simulink model "exampleModel_bus_axi_w_4ptavg"  (R2017b)
settings: Solver=VariableStepAuto  StartTime=0.0  StopTime=10e-5  RelTol=1e-3
PreLoadFcn:
  | setup
values from neighbouring files (symbols this model uses):
  axiClk = 156.25e6    (= 156250000)    [setup.m]    (also in setup_exampleModel_bus_axi_simulink.m; setup_exampleModel_bus_axi_simulink_lcls2.m; setup_lcls2_pcav.m; sysgen_signal.m)
  cav1p1_addr = 204    [setup_exampleModel_bus_axi_simulink.m]    (also in setup_exampleModel_bus_axi_simulink_lcls2.m; setup_lcls2_pcav.m; sysgen_signal.m)
  cav1p2_addr = cav1p1_addr * 2    (= 408)    [setup_exampleModel_bus_axi_simulink.m]    (also in setup_exampleModel_bus_axi_simulink_lcls2.m; setup_lcls2_pcav.m; sysgen_signal.m)
  cav2p1_addr = cav1p1_addr * 3    (= 612)    [setup_exampleModel_bus_axi_simulink.m]    (also in setup_exampleModel_bus_axi_simulink_lcls2.m; setup_lcls2_pcav.m; sysgen_signal.m)
  cav2p2_addr = cav1p1_addr * 4    (= 816)    [setup_exampleModel_bus_axi_simulink.m]    (also in setup_exampleModel_bus_axi_simulink_lcls2.m; setup_lcls2_pcav.m; sysgen_signal.m)
  Fadc = Fs/interleavedChannels    (= 29750000)    [setup.m]    (also in setup_exampleModel_bus_axi_simulink.m = 357000000; setup_exampleModel_bus_axi_simulink_lcls2.m = 351000000; setup_lcls2_pcav.m = 357000000; sysgen_signal.m = 357000000)
  fir_lpf = fir1(15, w_lpf)    [setup_exampleModel_bus_axi_simulink.m]    (also in setup_exampleModel_bus_axi_simulink_lcls2.m; setup_lcls2_pcav.m)
  Fproc = 204e6    (= 204000000)    [setup_exampleModel_bus_axi_simulink.m]    (also in setup_exampleModel_bus_axi_simulink_lcls2.m = 200571400; setup_lcls2_pcav.m; sysgen_signal.m)
  Fsig = Fproc/12    (= 17000000)    [setup_exampleModel_bus_axi_simulink.m]    (also in setup_exampleModel_bus_axi_simulink_lcls2.m = 16714283.3333; setup_lcls2_pcav.m)
  Tadc = 1/fadc    (= 2.80112044818e-09)    [cavity_signal.m]    (also in setup_exampleModel_bus_axi_simulink.m; setup_exampleModel_bus_axi_simulink_lcls2.m = 2.849002849e-09; setup_lcls2_pcav.m; setup_pcav_simulink.m)
undefined symbols (not defined in the file or in its folder): AXI4, Lite
libraries: xbsIndex_r4 x2870, llrf_lib x10, simulink x3
(part 8 of 15)

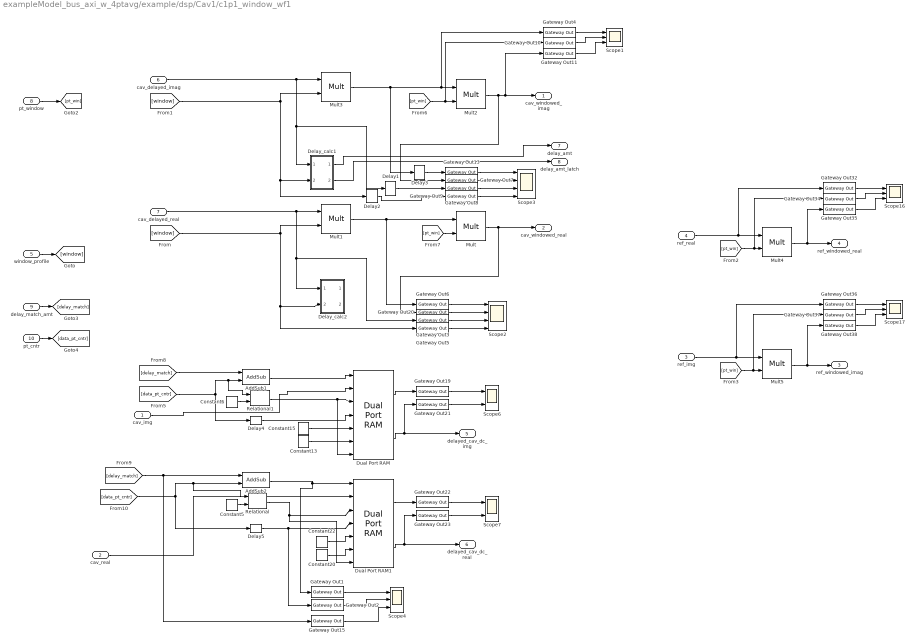
== system exampleModel_bus_axi_w_4ptavg/example/dsp/Cav1/c1p1_window_wf1  ==
  cav_img : Inport
  cav_real : Inport  Port=2
  ref_img : Inport  Port=3
  ref_real : Inport  Port=4
  window_profile : Inport  Port=5
  cav_delayed_imag : Inport  Port=6
  cav_delayed_real : Inport  Port=7
  pt_window : Inport  Port=8
  delay_match_amt : Inport  Port=9
  pt_cntr : Inport  Port=10
  AddSub1 : xbsIndex_r4/AddSub  mode=Addition  use_carryin=off  use_carryout=off  en=off  latency=1  precision=User Defined  arith_type=Unsigned  n_bits=16  bin_pt=0  quantization=Truncate  overflow=Wrap  use_behavioral_HDL=off  hw_selection=Fabric  pipelined=off  dbl_ovrd=off  block_type=addsub
  AddSub2 : xbsIndex_r4/AddSub  mode=Addition  use_carryin=off  use_carryout=off  en=off  latency=1  precision=User Defined  arith_type=Unsigned  n_bits=16  bin_pt=0  quantization=Truncate  overflow=Wrap  use_behavioral_HDL=off  hw_selection=Fabric  pipelined=off  dbl_ovrd=off  block_type=addsub
  Constant13 : xbsIndex_r4/Constant  const=1  gui_display_data_type=Boolean  arith_type=Boolean  n_bits=16  bin_pt=14  preci_type=Single  exp_width=8  frac_width=24  explicit_period=off  period=1  equ=P=C  opselect=C  inp2=PCIN>>17  opr=+  inp1=P  carry=CIN  dbl_ovrd=off  block_type=constant
  Constant{5..6,15,22} (4 alike) : xbsIndex_r4/Constant  const=0  gui_display_data_type=Fixed-point  arith_type=Signed (2's comp)  n_bits=18  bin_pt=16  preci_type=Single  exp_width=8  frac_width=24  explicit_period=off  period=1  equ=P=C  opselect=C  inp2=PCIN>>17  opr=+  inp1=P  carry=CIN  dbl_ovrd=off  block_type=constant
  Constant20 : xbsIndex_r4/Constant  const=1  gui_display_data_type=Boolean  arith_type=Boolean  n_bits=16  bin_pt=14  preci_type=Single  exp_width=8  frac_width=24  explicit_period=off  period=1  equ=P=C  opselect=C  inp2=PCIN>>17  opr=+  inp1=P  carry=CIN  dbl_ovrd=off  block_type=constant
  Delay1 : xbsIndex_r4/Delay  rst=off  infoeditControl=Selection of Reset will increase slice count due to use of real FFs and instead of SRLs  en=off  latency=6  reg_retiming=off  dbl_ovrd=off  block_type=delay
  Delay2 : xbsIndex_r4/Delay  rst=off  infoeditControl=Selection of Reset will increase slice count due to use of real FFs and instead of SRLs  en=off  latency=6  reg_retiming=off  dbl_ovrd=off  block_type=delay
  Delay3 : xbsIndex_r4/Delay  rst=off  infoeditControl=Selection of Reset will increase slice count due to use of real FFs and instead of SRLs  en=off  latency=3  reg_retiming=off  dbl_ovrd=off  block_type=delay
  Delay4 : xbsIndex_r4/Delay  rst=off  infoeditControl=Selection of Reset will increase slice count due to use of real FFs and instead of SRLs  en=off  latency=1  reg_retiming=off  dbl_ovrd=off  block_type=delay
  Delay5 : xbsIndex_r4/Delay  rst=off  infoeditControl=Selection of Reset will increase slice count due to use of real FFs and instead of SRLs  en=off  latency=1  reg_retiming=off  dbl_ovrd=off  block_type=delay
  Delay_calc1 : Subsystem
  Delay_calc2 : Subsystem
  Dual Port RAM : xbsIndex_r4/Dual Port RAM  depth=2^16  initVector=zeros(2^16,1)  distributed_mem=Block RAM  init_a=0  init_b=0  rst_a=off  rst_b=off  en_a=off  en_b=on  latency=1  write_mode_A=Read After Write  write_mode_B=Read Before Write  optimize=Area  dbl_ovrd=off  block_type=dpram
  Dual Port RAM1 : xbsIndex_r4/Dual Port RAM  depth=2^16  initVector=zeros(2^16,1)  distributed_mem=Block RAM  init_a=0  init_b=0  rst_a=off  rst_b=off  en_a=off  en_b=on  latency=1  write_mode_A=Read After Write  write_mode_B=Read Before Write  optimize=Area  dbl_ovrd=off  block_type=dpram
  Gateway Out{1..3,5..9,13,15,19..23} (15 alike) : xbsIndex_r4/Gateway Out  inherit_from_input=off  hdl_port=off  rows=1  columns=1  UseAsDAC=off  DACChannel='1'  interface=None  automatic_assignment=on  address_offset=hex2dec('00')  intf_name=''  intf_description=''  timing_constraint=None  locs_specified=off  LOCs={}  io_standard={}  block_type=gatewayout
  Gateway Out{4,10..11,32,34..38} (9 alike) : xbsIndex_r4/Gateway Out  inherit_from_input=off  hdl_port=on  rows=1  columns=1  UseAsDAC=off  DACChannel='1'  interface=None  automatic_assignment=on  address_offset=hex2dec('00')  intf_name=''  intf_description=''  timing_constraint=None  locs_specified=off  LOCs={}  io_standard={}  block_type=gatewayout
  Mult{,2,4..5} (4 alike) : xbsIndex_r4/Mult  precision=User Defined  arith_type="Signed  (2's comp)"  n_bits=18  bin_pt=16  quantization=Truncate  overflow=Wrap  en=off  latency=3  use_behavioral_HDL=off  opt=Speed  use_embedded=on  optimum_pipeline=off  pipeline=on  dbl_ovrd=off  use_rpm=on  placement_style=Triangular  block_type=mult
  Mult1 : xbsIndex_r4/Mult  precision=User Defined  arith_type="Signed  (2's comp)"  n_bits=18  bin_pt=17  quantization=Truncate  overflow=Wrap  en=off  latency=3  use_behavioral_HDL=off  opt=Speed  use_embedded=on  optimum_pipeline=off  pipeline=on  dbl_ovrd=off  use_rpm=on  placement_style=Triangular  block_type=mult
  Mult3 : xbsIndex_r4/Mult  precision=User Defined  arith_type="Signed  (2's comp)"  n_bits=18  bin_pt=17  quantization=Truncate  overflow=Wrap  en=off  latency=3  use_behavioral_HDL=off  opt=Speed  use_embedded=on  optimum_pipeline=off  pipeline=on  dbl_ovrd=off  use_rpm=on  placement_style=Triangular  block_type=mult
  Relational : xbsIndex_r4/Relational  mode=a>b  op_type=Bool  en=off  latency=1  dbl_ovrd=off  block_type=relational
  Relational1 : xbsIndex_r4/Relational  mode=a>b  op_type=Bool  en=off  latency=1  dbl_ovrd=off  block_type=relational
  Scope{1,4,16..17} (4 alike) : Scope  NumInputPorts=3
  Scope2 : Scope  NumInputPorts=4
  Scope3 : Scope  NumInputPorts=4
  Scope6 : Scope  NumInputPorts=2
  Scope7 : Scope  NumInputPorts=2
  cav_windowed_imag : Outport
  cav_windowed_real : Outport  Port=2
  ref_windowed_imag : Outport  Port=3
  ref_windowed_real : Outport  Port=4
  delayed_cav_dc_img : Outport  Port=5
  delayed_cav_dc_real : Outport  Port=6
  delay_amt : Outport  Port=7
  delay_amt_latch : Outport  Port=8
  wires:
  cav_real/1 -> Dual Port RAM1/2
  Relational/1 -> Dual Port RAM1/7, Dual Port RAM1/3
  Mult2/1 -> Gateway Out11/1, cav_windowed_imag/1, Gateway Out7/1
  Gateway Out23/1 -> Scope7/2
  Gateway Out21/1 -> Scope6/2
  Dual Port RAM1/1 -> Gateway Out22/1
  [data_pt_cntr] -> Relational1/1, AddSub1/2, Delay4/1
  Constant15/1 -> Dual Port RAM/5
  Gateway Out20/1 -> Scope2/2
  AddSub1/1 -> Dual Port RAM/1
  [pt_win] -> Gateway Out10/1, Mult2/2
  Gateway Out8/1 -> Scope3/3
  Gateway Out3/1 -> Scope2/3
  Constant13/1 -> Dual Port RAM/6
  Mult/1 -> cav_windowed_real/1, Gateway Out20/1
  cav_delayed_imag/1 -> Mult3/1, Delay_calc1/1(wav), Delay1/1
  [delay_match] -> Gateway Out15/1, AddSub2/1
  Gateway Out19/1 -> Scope6/1
  Gateway Out9/1 -> Scope3/4
  [data_pt_cntr] -> Delay5/1, Relational/1, AddSub2/2
  Dual Port RAM/1 -> Gateway Out19/1
  Gateway Out22/1 -> Scope7/1
  [window] -> Delay_calc1/2(win), Delay2/1, Mult3/2
  [window] -> Mult1/2, Delay_calc2/2(win), Gateway Out5/1
  cav_delayed_real/1 -> Delay_calc2/1(wav), Gateway Out3/1, Mult1/1
  Constant20/1 -> Dual Port RAM1/6
  Mult1/1 -> Gateway Out6/1, Mult/1
  Constant22/1 -> Dual Port RAM1/5
  Gateway Out6/1 -> Scope2/1
  Gateway Out13/1 -> Scope3/1
  [delay_match] -> AddSub1/1
  Gateway Out5/1 -> Scope2/4
  Gateway Out7/1 -> Scope3/2
  [pt_win] -> Mult/2
  Gateway Out35/1 -> Scope16/3
  ref_img/1 -> Gateway Out36/1, Mult5/1
  [pt_win] -> Gateway Out37/1, Mult5/2
  [pt_win] -> Gateway Out34/1, Mult4/2
  ref_real/1 -> Gateway Out32/1, Mult4/1
  Mult5/1 -> ref_windowed_imag/1, Gateway Out38/1
  Gateway Out38/1 -> Scope17/3
  Gateway Out36/1 -> Scope17/1
  Gateway Out32/1 -> Scope16/1
  Gateway Out34/1 -> Scope16/2
  Mult4/1 -> ref_windowed_real/1, Gateway Out35/1
  Gateway Out37/1 -> Scope17/2
  window_profile/1 -> [window]
  Delay_calc1/1(delay_amt) -> delay_amt/1
  pt_window/1 -> [pt_win]
  delay_match_amt/1 -> [delay_match]
  pt_cntr/1 -> [data_pt_cntr]
  Mult3/1 -> Delay3/1, Gateway Out4/1, Mult2/1
  Delay1/1 -> Gateway Out8/1
  Delay2/1 -> Gateway Out9/1
  Delay3/1 -> Gateway Out13/1
  Delay_calc1/2(delay_fb_latch) -> delay_amt_latch/1
  Gateway Out1/1 -> Scope4/1
  Gateway Out2/1 -> Scope4/2
  AddSub2/1 -> Gateway Out1/1, Dual Port RAM1/1
  cav_img/1 -> Dual Port RAM/2
  Delay4/1 -> Dual Port RAM/4
  Gateway Out15/1 -> Scope4/3
  Delay5/1 -> Gateway Out2/1, Dual Port RAM1/4
  Dual Port RAM1/2 -> delayed_cav_dc_real/1, Gateway Out23/1
  Dual Port RAM/2 -> delayed_cav_dc_img/1, Gateway Out21/1
  Constant5/1 -> Relational/2
  Constant6/1 -> Relational1/2
  Relational1/1 -> Dual Port RAM/7, Dual Port RAM/3
  Gateway Out10/1 -> Scope1/2
  Gateway Out4/1 -> Scope1/1
  Gateway Out11/1 -> Scope1/3

== system exampleModel_bus_axi_w_4ptavg/example/dsp/Cav1/c1p2_freq_err_module ==
  imag : Inport
  real : Inport  Port=2
  flo_window : Inport  Port=3
  reset : Inport  Port=4
  CORDIC 6.0 2 : xbsIndex_r4/CORDIC 6.0   functional_selection=Translate  architectural_configuration=Parallel  pipelining_mode=Maximum  data_format=SignedFraction  phase_format=Radians  input_width=18  output_width=18  round_mode=Truncate  iterations=0  precision=0  compensation_scaling=No_Scale_Compensation  coarse_rotation=on  aclken=off  aresetn=off  out_tready=off  cartesian_has_tuser=off  cartesian_has_tlast=off  cartesian_tuser_width=1  phase_has_tuser=off  phase_has_tlast=off  phase_tuser_width=1  out_tlast_behv=Null  flow_control=NonBlocking  optimize_goal=Resources  trim_axipin_name=on  simulation_type=hybrid_sim  simulation_model=sysgen:cordic_v6_0  data_path_portlist={'s_axis_cartesian_tdata_imag', 's_axis_cartesian_tdata_real', 's_axis_phase_tdata_phase', 'm_axis_dout_tdata_imag', 'm_axis_dout_tdata_real', 'm_axis_dout_tdata_phase','m_axis_dout_tdata'}  ip_name=CORDIC  ip_version=6.0  dsptool_ready=true  ipcore_usecache=true  ipcore_useipmodelcache=true  wrapper_available=true  port_translation_map={ 'aclken' => 'en', 'aresetn' => 'rst' }  block_type=cordic_v6_0
      settings: infoedit=CORDIC 6.0
  Clock Enable Probe4 : xbsIndex_r4/Clock Enable Probe  inherit_constraints=on  block_type=ceprobe
      settings: infoedit="Clock enable extractor.  Produces a Boolean output that mirrors the hardware clock enable associated with the input sample rate.<br><br>Hardware notes: in hardware this block costs nothing."
  Down Sample5 : xbsIndex_r4/Down Sample  sample_ratio=12  sample_phase="Last Value of Frame  (most efficient)"  en=off  rst=off  latency=1  dbl_ovrd=off  block_type=dsamp
  Gateway Out{1..3,38,41,53} (6 alike) : xbsIndex_r4/Gateway Out  inherit_from_input=off  hdl_port=off  rows=1  columns=1  UseAsDAC=off  DACChannel='1'  interface=None  automatic_assignment=on  address_offset=hex2dec('00')  intf_name=''  intf_description=''  timing_constraint=None  locs_specified=off  LOCs={}  io_standard={}  block_type=gatewayout
  Gateway Out44 : xbsIndex_r4/Gateway Out  inherit_from_input=off  hdl_port=on  rows=1  columns=1  UseAsDAC=off  DACChannel='1'  interface=None  automatic_assignment=on  address_offset=hex2dec('00')  intf_name=''  intf_description=''  timing_constraint=None  locs_specified=off  LOCs={}  io_standard={}  block_type=gatewayout
  Gateway Out46 : xbsIndex_r4/Gateway Out  inherit_from_input=off  hdl_port=on  rows=1  columns=1  UseAsDAC=off  DACChannel='1'  interface=None  automatic_assignment=on  address_offset=hex2dec('00')  intf_name=''  intf_description=''  timing_constraint=None  locs_specified=off  LOCs={}  io_standard={}  block_type=gatewayout
  Mult3 : xbsIndex_r4/Mult  precision=User Defined  arith_type="Signed  (2's comp)"  n_bits=18  bin_pt=15  quantization=Truncate  overflow=Saturate  en=off  latency=3  use_behavioral_HDL=off  opt=Speed  use_embedded=on  optimum_pipeline=off  pipeline=on  dbl_ovrd=off  use_rpm=on  placement_style=Triangular  block_type=mult
  Scope1 : Scope  NumInputPorts=3
  Scope21 : Scope  NumInputPorts=3
  Scope22 : Scope  NumInputPorts=2
  freq_err1 : Subsystem
  NCO_err_fb : Outport
  freq_err : Outport  Port=2
  wires:
  [c1p2_pt_cntr] -> Gateway Out41/1
  Down Sample5/1 -> CORDIC 6.0 2/1
  Gateway Out38/1 -> Scope21/2
  reset/1 -> freq_err1/3(reset)
  Clock Enable Probe4/1 -> Down Sample5/1
  CORDIC 6.0 2/2 -> freq_err1/1(raw_phase), Gateway Out38/1
  real/1 -> CORDIC 6.0 2/3, Gateway Out44/1
  imag/1 -> CORDIC 6.0 2/2, Clock Enable Probe4/1, Gateway Out46/1
  flo_window/1 -> Gateway Out2/1, Mult3/2, freq_err1/2(window)
  Gateway Out44/1 -> Scope22/2
  Gateway Out53/1 -> Scope21/1
  Gateway Out41/1 -> Scope21/3
  freq_err1/1(NCO_err) -> NCO_err_fb/1
  Gateway Out46/1 -> Scope22/1
  freq_err1/2(freq_err) -> freq_err/1
  Mult3/1 -> Gateway Out1/1
  Gateway Out1/1 -> Scope1/3
  Gateway Out3/1 -> Scope1/1
  Gateway Out2/1 -> Scope1/2
  CORDIC 6.0 2/3 -> Gateway Out3/1, Mult3/1, Gateway Out53/1

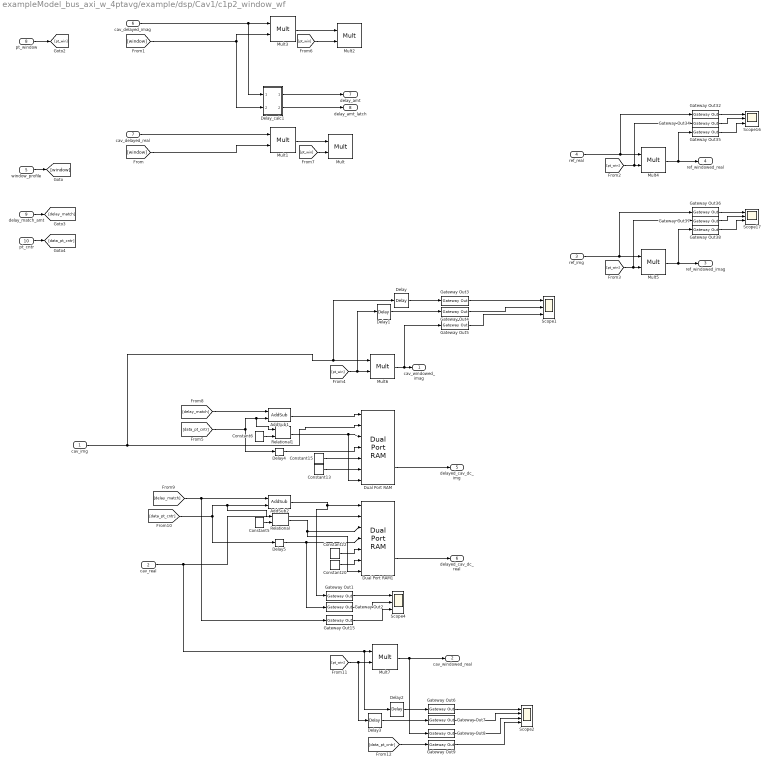
== system exampleModel_bus_axi_w_4ptavg/example/dsp/Cav1/c1p2_window_wf ==
  cav_img : Inport
  cav_real : Inport  Port=2
  ref_img : Inport  Port=3
  ref_real : Inport  Port=4
  window_profile : Inport  Port=5
  cav_delayed_imag : Inport  Port=6
  cav_delayed_real : Inport  Port=7
  pt_window : Inport  Port=8
  delay_match_amt : Inport  Port=9
  pt_cntr : Inport  Port=10
  AddSub1 : xbsIndex_r4/AddSub  mode=Addition  use_carryin=off  use_carryout=off  en=off  latency=1  precision=User Defined  arith_type=Unsigned  n_bits=16  bin_pt=0  quantization=Truncate  overflow=Wrap  use_behavioral_HDL=off  hw_selection=Fabric  pipelined=off  dbl_ovrd=off  block_type=addsub
  AddSub2 : xbsIndex_r4/AddSub  mode=Addition  use_carryin=off  use_carryout=off  en=off  latency=1  precision=User Defined  arith_type=Unsigned  n_bits=16  bin_pt=0  quantization=Truncate  overflow=Wrap  use_behavioral_HDL=off  hw_selection=Fabric  pipelined=off  dbl_ovrd=off  block_type=addsub
  Constant13 : xbsIndex_r4/Constant  const=1  gui_display_data_type=Boolean  arith_type=Boolean  n_bits=16  bin_pt=14  preci_type=Single  exp_width=8  frac_width=24  explicit_period=off  period=1  equ=P=C  opselect=C  inp2=PCIN>>17  opr=+  inp1=P  carry=CIN  dbl_ovrd=off  block_type=constant
  Constant{5..6,15,22} (4 alike) : xbsIndex_r4/Constant  const=0  gui_display_data_type=Fixed-point  arith_type=Signed (2's comp)  n_bits=18  bin_pt=16  preci_type=Single  exp_width=8  frac_width=24  explicit_period=off  period=1  equ=P=C  opselect=C  inp2=PCIN>>17  opr=+  inp1=P  carry=CIN  dbl_ovrd=off  block_type=constant
  Constant20 : xbsIndex_r4/Constant  const=1  gui_display_data_type=Boolean  arith_type=Boolean  n_bits=16  bin_pt=14  preci_type=Single  exp_width=8  frac_width=24  explicit_period=off  period=1  equ=P=C  opselect=C  inp2=PCIN>>17  opr=+  inp1=P  carry=CIN  dbl_ovrd=off  block_type=constant
  Delay{,1..3} (4 alike) : xbsIndex_r4/Delay  rst=off  infoeditControl=Selection of Reset will increase slice count due to use of real FFs and instead of SRLs  en=off  latency=3  reg_retiming=off  dbl_ovrd=off  block_type=delay
  Delay4 : xbsIndex_r4/Delay  rst=off  infoeditControl=Selection of Reset will increase slice count due to use of real FFs and instead of SRLs  en=off  latency=1  reg_retiming=off  dbl_ovrd=off  block_type=delay
  Delay5 : xbsIndex_r4/Delay  rst=off  infoeditControl=Selection of Reset will increase slice count due to use of real FFs and instead of SRLs  en=off  latency=1  reg_retiming=off  dbl_ovrd=off  block_type=delay
  Delay_calc1 : Subsystem
  Dual Port RAM : xbsIndex_r4/Dual Port RAM  depth=2^16  initVector=zeros(2^16,1)  distributed_mem=Block RAM  init_a=0  init_b=0  rst_a=off  rst_b=off  en_a=off  en_b=on  latency=1  write_mode_A=Read After Write  write_mode_B=Read Before Write  optimize=Area  dbl_ovrd=off  block_type=dpram
  Dual Port RAM1 : xbsIndex_r4/Dual Port RAM  depth=2^16  initVector=zeros(2^16,1)  distributed_mem=Block RAM  init_a=0  init_b=0  rst_a=off  rst_b=off  en_a=off  en_b=on  latency=1  write_mode_A=Read After Write  write_mode_B=Read Before Write  optimize=Area  dbl_ovrd=off  block_type=dpram
  Gateway Out{1..9,15} (10 alike) : xbsIndex_r4/Gateway Out  inherit_from_input=off  hdl_port=off  rows=1  columns=1  UseAsDAC=off  DACChannel='1'  interface=None  automatic_assignment=on  address_offset=hex2dec('00')  intf_name=''  intf_description=''  timing_constraint=None  locs_specified=off  LOCs={}  io_standard={}  block_type=gatewayout
  Gateway Out{32,34..38} (6 alike) : xbsIndex_r4/Gateway Out  inherit_from_input=off  hdl_port=on  rows=1  columns=1  UseAsDAC=off  DACChannel='1'  interface=None  automatic_assignment=on  address_offset=hex2dec('00')  intf_name=''  intf_description=''  timing_constraint=None  locs_specified=off  LOCs={}  io_standard={}  block_type=gatewayout
  Mult{,2,4..7} (6 alike) : xbsIndex_r4/Mult  precision=User Defined  arith_type="Signed  (2's comp)"  n_bits=18  bin_pt=16  quantization=Truncate  overflow=Wrap  en=off  latency=3  use_behavioral_HDL=off  opt=Speed  use_embedded=on  optimum_pipeline=off  pipeline=on  dbl_ovrd=off  use_rpm=on  placement_style=Triangular  block_type=mult
  Mult1 : xbsIndex_r4/Mult  precision=User Defined  arith_type="Signed  (2's comp)"  n_bits=18  bin_pt=17  quantization=Truncate  overflow=Wrap  en=off  latency=3  use_behavioral_HDL=off  opt=Speed  use_embedded=on  optimum_pipeline=off  pipeline=on  dbl_ovrd=off  use_rpm=on  placement_style=Triangular  block_type=mult
  Mult3 : xbsIndex_r4/Mult  precision=Full  arith_type="Signed  (2's comp)"  n_bits=18  bin_pt=17  quantization=Truncate  overflow=Wrap  en=off  latency=3  use_behavioral_HDL=off  opt=Speed  use_embedded=on  optimum_pipeline=off  pipeline=on  dbl_ovrd=off  use_rpm=on  placement_style=Triangular  block_type=mult
  Relational : xbsIndex_r4/Relational  mode=a>b  op_type=Bool  en=off  latency=1  dbl_ovrd=off  block_type=relational
  Relational1 : xbsIndex_r4/Relational  mode=a>b  op_type=Bool  en=off  latency=1  dbl_ovrd=off  block_type=relational
  Scope{1,4,16..17} (4 alike) : Scope  NumInputPorts=3
  Scope2 : Scope  NumInputPorts=4
  cav_windowed_imag : Outport
  cav_windowed_real : Outport  Port=2
  ref_windowed_imag : Outport  Port=3
  ref_windowed_real : Outport  Port=4
  delayed_cav_dc_img : Outport  Port=5
  delayed_cav_dc_real : Outport  Port=6
  delay_amt : Outport  Port=7
  delay_amt_latch : Outport  Port=8
  wires:
  Relational/1 -> Dual Port RAM1/7, Dual Port RAM1/3
  [data_pt_cntr] -> Relational1/1, AddSub1/2, Delay4/1
  Constant15/1 -> Dual Port RAM/5
  AddSub1/1 -> Dual Port RAM/1
  [pt_win] -> Mult2/2
  Constant13/1 -> Dual Port RAM/6
  cav_delayed_imag/1 -> Mult3/1, Delay_calc1/1(wav)
  [delay_match] -> Gateway Out15/1, AddSub2/1
  [data_pt_cntr] -> Delay5/1, Relational/1, AddSub2/2
  [window] -> Delay_calc1/2(win), Mult3/2
  [window] -> Mult1/2
  cav_delayed_real/1 -> Mult1/1
  Constant20/1 -> Dual Port RAM1/6
  Mult1/1 -> Mult/1
  Constant22/1 -> Dual Port RAM1/5
  [delay_match] -> AddSub1/1
  [pt_win] -> Mult/2
  Gateway Out35/1 -> Scope16/3
  ref_img/1 -> Gateway Out36/1, Mult5/1
  [pt_win] -> Gateway Out37/1, Mult5/2
  [pt_win] -> Gateway Out34/1, Mult4/2
  ref_real/1 -> Gateway Out32/1, Mult4/1
  Mult5/1 -> ref_windowed_imag/1, Gateway Out38/1
  Gateway Out38/1 -> Scope17/3
  Gateway Out36/1 -> Scope17/1
  Gateway Out32/1 -> Scope16/1
  Gateway Out34/1 -> Scope16/2
  Mult4/1 -> ref_windowed_real/1, Gateway Out35/1
  Gateway Out37/1 -> Scope17/2
  window_profile/1 -> [window]
  Delay_calc1/1(delay_amt) -> delay_amt/1
  pt_window/1 -> [pt_win]
  delay_match_amt/1 -> [delay_match]
  pt_cntr/1 -> [data_pt_cntr]
  Mult3/1 -> Mult2/1
  Delay_calc1/2(delay_fb_latch) -> delay_amt_latch/1
  Gateway Out1/1 -> Scope4/1
  Gateway Out2/1 -> Scope4/2
  AddSub2/1 -> Gateway Out1/1, Dual Port RAM1/1
  Delay4/1 -> Dual Port RAM/4
  Gateway Out15/1 -> Scope4/3
  Delay5/1 -> Gateway Out2/1, Dual Port RAM1/4
  Dual Port RAM1/2 -> delayed_cav_dc_real/1
  Dual Port RAM/2 -> delayed_cav_dc_img/1
  Constant5/1 -> Relational/2
  Constant6/1 -> Relational1/2
  Relational1/1 -> Dual Port RAM/7, Dual Port RAM/3
  [pt_win] -> Delay1/1, Mult6/2
  [pt_win] -> Delay3/1, Mult7/2
  Mult7/1 -> Gateway Out8/1, cav_windowed_real/1
  cav_real/1 -> Delay2/1, Mult7/1, Dual Port RAM1/2
  cav_img/1 -> Dual Port RAM/2, Delay/1, Mult6/1
  Mult6/1 -> Gateway Out5/1, cav_windowed_imag/1
  Gateway Out3/1 -> Scope1/1
  Gateway Out4/1 -> Scope1/2
  Gateway Out5/1 -> Scope1/3
  Gateway Out8/1 -> Scope2/3
  Gateway Out6/1 -> Scope2/1
  Gateway Out7/1 -> Scope2/2
  [data_pt_cntr] -> Gateway Out9/1
  Gateway Out9/1 -> Scope2/4
  Delay/1 -> Gateway Out3/1
  Delay1/1 -> Gateway Out4/1
  Delay2/1 -> Gateway Out6/1
  Delay3/1 -> Gateway Out7/1

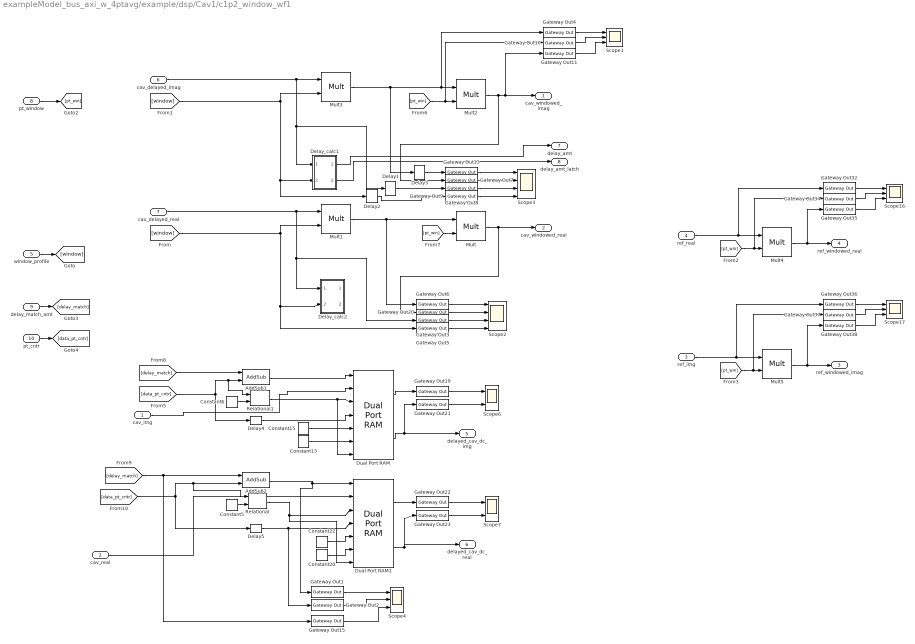
== system exampleModel_bus_axi_w_4ptavg/example/dsp/Cav1/c1p2_window_wf1 ==
  cav_img : Inport
  cav_real : Inport  Port=2
  ref_img : Inport  Port=3
  ref_real : Inport  Port=4
  window_profile : Inport  Port=5
  cav_delayed_imag : Inport  Port=6
  cav_delayed_real : Inport  Port=7
  pt_window : Inport  Port=8
  delay_match_amt : Inport  Port=9
  pt_cntr : Inport  Port=10
  AddSub1 : xbsIndex_r4/AddSub  mode=Addition  use_carryin=off  use_carryout=off  en=off  latency=1  precision=User Defined  arith_type=Unsigned  n_bits=16  bin_pt=0  quantization=Truncate  overflow=Wrap  use_behavioral_HDL=off  hw_selection=Fabric  pipelined=off  dbl_ovrd=off  block_type=addsub
  AddSub2 : xbsIndex_r4/AddSub  mode=Addition  use_carryin=off  use_carryout=off  en=off  latency=1  precision=User Defined  arith_type=Unsigned  n_bits=16  bin_pt=0  quantization=Truncate  overflow=Wrap  use_behavioral_HDL=off  hw_selection=Fabric  pipelined=off  dbl_ovrd=off  block_type=addsub
  Constant13 : xbsIndex_r4/Constant  const=1  gui_display_data_type=Boolean  arith_type=Boolean  n_bits=16  bin_pt=14  preci_type=Single  exp_width=8  frac_width=24  explicit_period=off  period=1  equ=P=C  opselect=C  inp2=PCIN>>17  opr=+  inp1=P  carry=CIN  dbl_ovrd=off  block_type=constant
  Constant{5..6,15,22} (4 alike) : xbsIndex_r4/Constant  const=0  gui_display_data_type=Fixed-point  arith_type=Signed (2's comp)  n_bits=18  bin_pt=16  preci_type=Single  exp_width=8  frac_width=24  explicit_period=off  period=1  equ=P=C  opselect=C  inp2=PCIN>>17  opr=+  inp1=P  carry=CIN  dbl_ovrd=off  block_type=constant
  Constant20 : xbsIndex_r4/Constant  const=1  gui_display_data_type=Boolean  arith_type=Boolean  n_bits=16  bin_pt=14  preci_type=Single  exp_width=8  frac_width=24  explicit_period=off  period=1  equ=P=C  opselect=C  inp2=PCIN>>17  opr=+  inp1=P  carry=CIN  dbl_ovrd=off  block_type=constant
  Delay1 : xbsIndex_r4/Delay  rst=off  infoeditControl=Selection of Reset will increase slice count due to use of real FFs and instead of SRLs  en=off  latency=6  reg_retiming=off  dbl_ovrd=off  block_type=delay
  Delay2 : xbsIndex_r4/Delay  rst=off  infoeditControl=Selection of Reset will increase slice count due to use of real FFs and instead of SRLs  en=off  latency=6  reg_retiming=off  dbl_ovrd=off  block_type=delay
  Delay3 : xbsIndex_r4/Delay  rst=off  infoeditControl=Selection of Reset will increase slice count due to use of real FFs and instead of SRLs  en=off  latency=3  reg_retiming=off  dbl_ovrd=off  block_type=delay
  Delay4 : xbsIndex_r4/Delay  rst=off  infoeditControl=Selection of Reset will increase slice count due to use of real FFs and instead of SRLs  en=off  latency=1  reg_retiming=off  dbl_ovrd=off  block_type=delay
  Delay5 : xbsIndex_r4/Delay  rst=off  infoeditControl=Selection of Reset will increase slice count due to use of real FFs and instead of SRLs  en=off  latency=1  reg_retiming=off  dbl_ovrd=off  block_type=delay
  Delay_calc1 : Subsystem
  Delay_calc2 : Subsystem
  Dual Port RAM : xbsIndex_r4/Dual Port RAM  depth=2^16  initVector=zeros(2^16,1)  distributed_mem=Block RAM  init_a=0  init_b=0  rst_a=off  rst_b=off  en_a=off  en_b=on  latency=1  write_mode_A=Read After Write  write_mode_B=Read Before Write  optimize=Area  dbl_ovrd=off  block_type=dpram
  Dual Port RAM1 : xbsIndex_r4/Dual Port RAM  depth=2^16  initVector=zeros(2^16,1)  distributed_mem=Block RAM  init_a=0  init_b=0  rst_a=off  rst_b=off  en_a=off  en_b=on  latency=1  write_mode_A=Read After Write  write_mode_B=Read Before Write  optimize=Area  dbl_ovrd=off  block_type=dpram
  Gateway Out{1..3,5..9,13,15,19..23} (15 alike) : xbsIndex_r4/Gateway Out  inherit_from_input=off  hdl_port=off  rows=1  columns=1  UseAsDAC=off  DACChannel='1'  interface=None  automatic_assignment=on  address_offset=hex2dec('00')  intf_name=''  intf_description=''  timing_constraint=None  locs_specified=off  LOCs={}  io_standard={}  block_type=gatewayout
  Gateway Out{4,10..11,32,34..38} (9 alike) : xbsIndex_r4/Gateway Out  inherit_from_input=off  hdl_port=on  rows=1  columns=1  UseAsDAC=off  DACChannel='1'  interface=None  automatic_assignment=on  address_offset=hex2dec('00')  intf_name=''  intf_description=''  timing_constraint=None  locs_specified=off  LOCs={}  io_standard={}  block_type=gatewayout
  Mult{,2,4..5} (4 alike) : xbsIndex_r4/Mult  precision=User Defined  arith_type="Signed  (2's comp)"  n_bits=18  bin_pt=16  quantization=Truncate  overflow=Wrap  en=off  latency=3  use_behavioral_HDL=off  opt=Speed  use_embedded=on  optimum_pipeline=off  pipeline=on  dbl_ovrd=off  use_rpm=on  placement_style=Triangular  block_type=mult
  Mult1 : xbsIndex_r4/Mult  precision=User Defined  arith_type="Signed  (2's comp)"  n_bits=18  bin_pt=17  quantization=Truncate  overflow=Wrap  en=off  latency=3  use_behavioral_HDL=off  opt=Speed  use_embedded=on  optimum_pipeline=off  pipeline=on  dbl_ovrd=off  use_rpm=on  placement_style=Triangular  block_type=mult
  Mult3 : xbsIndex_r4/Mult  precision=Full  arith_type="Signed  (2's comp)"  n_bits=18  bin_pt=17  quantization=Truncate  overflow=Wrap  en=off  latency=3  use_behavioral_HDL=off  opt=Speed  use_embedded=on  optimum_pipeline=off  pipeline=on  dbl_ovrd=off  use_rpm=on  placement_style=Triangular  block_type=mult
  Relational : xbsIndex_r4/Relational  mode=a>b  op_type=Bool  en=off  latency=1  dbl_ovrd=off  block_type=relational
  Relational1 : xbsIndex_r4/Relational  mode=a>b  op_type=Bool  en=off  latency=1  dbl_ovrd=off  block_type=relational
  Scope{1,4,16..17} (4 alike) : Scope  NumInputPorts=3
  Scope2 : Scope  NumInputPorts=4
  Scope3 : Scope  NumInputPorts=4
  Scope6 : Scope  NumInputPorts=2
  Scope7 : Scope  NumInputPorts=2
  cav_windowed_imag : Outport
  cav_windowed_real : Outport  Port=2
  ref_windowed_imag : Outport  Port=3
  ref_windowed_real : Outport  Port=4
  delayed_cav_dc_img : Outport  Port=5
  delayed_cav_dc_real : Outport  Port=6
  delay_amt : Outport  Port=7
  delay_amt_latch : Outport  Port=8
  wires:
  Gateway Out11/1 -> Scope1/3
  Gateway Out4/1 -> Scope1/1
  Gateway Out10/1 -> Scope1/2
  Relational1/1 -> Dual Port RAM/3, Dual Port RAM/7
  Constant6/1 -> Relational1/2
  Constant5/1 -> Relational/2
  Dual Port RAM/2 -> Gateway Out21/1, delayed_cav_dc_img/1
  Dual Port RAM1/2 -> Gateway Out23/1, delayed_cav_dc_real/1
  Delay5/1 -> Dual Port RAM1/4, Gateway Out2/1
  Gateway Out15/1 -> Scope4/3
  Delay4/1 -> Dual Port RAM/4
  cav_img/1 -> Dual Port RAM/2
  AddSub2/1 -> Dual Port RAM1/1, Gateway Out1/1
  Gateway Out2/1 -> Scope4/2
  Gateway Out1/1 -> Scope4/1
  Delay_calc1/2(delay_fb_latch) -> delay_amt_latch/1
  Delay3/1 -> Gateway Out13/1
  Delay2/1 -> Gateway Out9/1
  Delay1/1 -> Gateway Out8/1
  Mult3/1 -> Mult2/1, Gateway Out4/1, Delay3/1
  pt_cntr/1 -> [data_pt_cntr]
  delay_match_amt/1 -> [delay_match]
  pt_window/1 -> [pt_win]
  Delay_calc1/1(delay_amt) -> delay_amt/1
  window_profile/1 -> [window]
  Gateway Out37/1 -> Scope17/2
  Mult4/1 -> Gateway Out35/1, ref_windowed_real/1
  Gateway Out34/1 -> Scope16/2
  Gateway Out32/1 -> Scope16/1
  Gateway Out36/1 -> Scope17/1
  Gateway Out38/1 -> Scope17/3
  Mult5/1 -> Gateway Out38/1, ref_windowed_imag/1
  ref_real/1 -> Mult4/1, Gateway Out32/1
  [pt_win] -> Mult4/2, Gateway Out34/1
  [pt_win] -> Mult5/2, Gateway Out37/1
  ref_img/1 -> Mult5/1, Gateway Out36/1
  Gateway Out35/1 -> Scope16/3
  [pt_win] -> Mult/2
  Gateway Out7/1 -> Scope3/2
  Gateway Out5/1 -> Scope2/4
  [delay_match] -> AddSub1/1
  Gateway Out13/1 -> Scope3/1
  Gateway Out6/1 -> Scope2/1
  Constant22/1 -> Dual Port RAM1/5
  Mult1/1 -> Mult/1, Gateway Out6/1
  Constant20/1 -> Dual Port RAM1/6
  cav_delayed_real/1 -> Mult1/1, Gateway Out3/1, Delay_calc2/1(wav)
  [window] -> Gateway Out5/1, Delay_calc2/2(win), Mult1/2
  [window] -> Mult3/2, Delay2/1, Delay_calc1/2(win)
  Gateway Out22/1 -> Scope7/1
  Dual Port RAM/1 -> Gateway Out19/1
  [data_pt_cntr] -> AddSub2/2, Relational/1, Delay5/1
  Gateway Out9/1 -> Scope3/4
  Gateway Out19/1 -> Scope6/1
  [delay_match] -> AddSub2/1, Gateway Out15/1
  cav_delayed_imag/1 -> Delay1/1, Delay_calc1/1(wav), Mult3/1
  Mult/1 -> Gateway Out20/1, cav_windowed_real/1
  Constant13/1 -> Dual Port RAM/6
  Gateway Out3/1 -> Scope2/3
  Gateway Out8/1 -> Scope3/3
  [pt_win] -> Mult2/2, Gateway Out10/1
  AddSub1/1 -> Dual Port RAM/1
  Gateway Out20/1 -> Scope2/2
  Constant15/1 -> Dual Port RAM/5
  [data_pt_cntr] -> Delay4/1, AddSub1/2, Relational1/1
  Dual Port RAM1/1 -> Gateway Out22/1
  Gateway Out21/1 -> Scope6/2
  Gateway Out23/1 -> Scope7/2
  Mult2/1 -> Gateway Out7/1, cav_windowed_imag/1, Gateway Out11/1
  Relational/1 -> Dual Port RAM1/3, Dual Port RAM1/7
  cav_real/1 -> Dual Port RAM1/2

== system exampleModel_bus_axi_w_4ptavg/example/dsp/Cav1/c1p2_windowing_func1 ==
  imag : Inport
  real : Inport  Port=2
  eval_window : Inport  Port=3
  "CORDIC 6.0 " : xbsIndex_r4/CORDIC 6.0   functional_selection=Translate  architectural_configuration=Parallel  pipelining_mode=Maximum  data_format=SignedFraction  phase_format=Scaled_Radians  input_width=18  output_width=18  round_mode=Truncate  iterations=0  precision=0  compensation_scaling=No_Scale_Compensation  coarse_rotation=on  aclken=off  aresetn=off  out_tready=off  cartesian_has_tuser=off  cartesian_has_tlast=off  cartesian_tuser_width=1  phase_has_tuser=off  phase_has_tlast=off  phase_tuser_width=1  out_tlast_behv=Null  flow_control=NonBlocking  optimize_goal=Resources  trim_axipin_name=on  simulation_type=hybrid_sim  simulation_model=sysgen:cordic_v6_0  data_path_portlist={'s_axis_cartesian_tdata_imag', 's_axis_cartesian_tdata_real', 's_axis_phase_tdata_phase', 'm_axis_dout_tdata_imag', 'm_axis_dout_tdata_real', 'm_axis_dout_tdata_phase','m_axis_dout_tdata'}  ip_name=CORDIC  ip_version=6.0  dsptool_ready=true  ipcore_usecache=true  ipcore_useipmodelcache=true  wrapper_available=true  port_translation_map={ 'aclken' => 'en', 'aresetn' => 'rst' }  block_type=cordic_v6_0
      settings: infoedit=CORDIC 6.0
  Gateway Out{1..5,7} (6 alike) : xbsIndex_r4/Gateway Out  inherit_from_input=off  hdl_port=off  rows=1  columns=1  UseAsDAC=off  DACChannel='1'  interface=None  automatic_assignment=on  address_offset=hex2dec('00')  intf_name=''  intf_description=''  timing_constraint=None  locs_specified=off  LOCs={}  io_standard={}  block_type=gatewayout
  Scope{1..4} (4 alike) : Scope  NumInputPorts=3
  four_point_avg : Subsystem
  Window_profile : Outport
  wires:
  four_point_avg/1(Out1) -> Gateway Out2/1, Window_profile/1
  "CORDIC 6.0 "/3 -> Gateway Out4/1, Gateway Out1/1, four_point_avg/1(In1)
  [cav1_p2_dc_tvalid] -> "CORDIC 6.0 "/1
  imag/1 -> "CORDIC 6.0 "/2
  real/1 -> "CORDIC 6.0 "/3
  Gateway Out5/1 -> Scope3/1, Scope2/2
  Gateway Out7/1 -> Scope4/2, Scope3/2
  [c1p2_pt_cntr] -> Gateway Out7/1
  eval_window/1 -> [window]
  "CORDIC 6.0 "/2 -> Gateway Out5/1
  Gateway Out4/1 -> Scope4/1, Scope2/1
  Gateway Out1/1 -> Scope1/1
  Gateway Out2/1 -> Scope1/2
  [window] -> Gateway Out3/1
  Gateway Out3/1 -> Scope4/3

== system exampleModel_bus_axi_w_4ptavg/example/dsp/Cav1/c1p2_windowing_func2 ==
  imag : Inport
  real : Inport  Port=2
  eval_window : Inport  Port=3
  "CORDIC 6.0 " : xbsIndex_r4/CORDIC 6.0   functional_selection=Translate  architectural_configuration=Parallel  pipelining_mode=Maximum  data_format=SignedFraction  phase_format=Scaled_Radians  input_width=18  output_width=18  round_mode=Truncate  iterations=0  precision=0  compensation_scaling=No_Scale_Compensation  coarse_rotation=on  aclken=off  aresetn=off  out_tready=off  cartesian_has_tuser=off  cartesian_has_tlast=off  cartesian_tuser_width=1  phase_has_tuser=off  phase_has_tlast=off  phase_tuser_width=1  out_tlast_behv=Null  flow_control=NonBlocking  optimize_goal=Resources  trim_axipin_name=on  simulation_type=hybrid_sim  simulation_model=sysgen:cordic_v6_0  data_path_portlist={'s_axis_cartesian_tdata_imag', 's_axis_cartesian_tdata_real', 's_axis_phase_tdata_phase', 'm_axis_dout_tdata_imag', 'm_axis_dout_tdata_real', 'm_axis_dout_tdata_phase','m_axis_dout_tdata'}  ip_name=CORDIC  ip_version=6.0  dsptool_ready=true  ipcore_usecache=true  ipcore_useipmodelcache=true  wrapper_available=true  port_translation_map={ 'aclken' => 'en', 'aresetn' => 'rst' }  block_type=cordic_v6_0
      settings: infoedit=CORDIC 6.0
  FIR Compiler 7.2 2 : xbsIndex_r4/FIR Compiler 7.2   coefficientvector=[fir_lpf]  coefficient_sets=1  coefficient_reload=off  filter_type=Single_Rate  rate_change_type=Integer  interpolation_rate=1  decimation_rate=1  zero_pack_factor=1  channel_sequence=Basic  number_channels=1  pattern_list='P4-0,P4-1,P4-2,P4-3,P4-4'  number_paths=1  ratespecification=Maximum_Possible  sampleperiod=12  hardwareoversamplingrate=1  coefficient_sign=Signed  quantization=Quantize_Only  coefficient_width=16  bestprecision=off  coefficient_fractional_bits=15  coefficient_structure=Inferred  output_rounding_mode=Truncate_LSBs  output_width=18  filter_architecture=Systolic_Multiply_Accumulate  optimization_goal=Area  optimization_list='None'  data_buffer_type=Automatic  coefficient_buffer_type=Automatic  input_buffer_type=Automatic  output_buffer_type=Automatic  preference_for_other_storage=Automatic  multi_column_support=Automatic  columnconfig='8'  inter_column_pipe_length=4  data_has_tlast=Not_Required  m_data_has_tready=off  s_data_has_fifo=off  s_data_has_tuser=Not_Required  m_data_has_tuser=Not_Required  s_config_sync_mode=On_Vector  s_config_method=Single  num_reload_slots=1  has_aclken=off  has_aresetn=off  infoeditControl=ARESETn must be asserted for a minimum of 2 cycles  reset_data_vector=on  trim_axipin_name=on  simulation_type=hybrid_sim  simulation_model=sysgen:xfirv7_2_cmodel  data_path_portlist={ 's_axis_data_tdata', 'm_axis_data_tdata' }  passband_min=0.0  passband_max=0.5  stopband_min=0.5  stopband_max=1.0  filter_selection=1  gui_behaviour='Sysgen_GUI'  data_sign=Signed  data_width=16  data_fractional_bits=0  data_tuser_width=1  wrapper_available=true  ip_wrap_arbitrary_binary_point=true  ip_name=FIR Compiler  ip_version=7.2  dsptool_ready=true  ipcore_usecache=true  ipcore_useipmodelcache=true  port_translation_map={ 'aclken' => 'en', 'aresetn' => 'rst' }  run_core_at_system_period=true  ipcore_xco_need_fpga_part=true  block_type=fir_compiler_v7_2
      settings: infoedit=Maximum Possible : Maximizes oversampling rate. Abstracted input handshake (no s_data_tvalid) and automatic rate propagation.<br>Hardware Oversampling Rate : Specifies oversampling rate relative to the input sample period. Abstracted input handshake (no s_data_tvalid) and automatic rate propagation.<br>Input/Output Sample Period : Specifies absolute oversampling rate. No input handshake abstraction (exposes s_data_tvalid) and no rate propagation.
  FIR Compiler 7.2 3 : xbsIndex_r4/FIR Compiler 7.2   coefficientvector=[fir_lpf]  coefficient_sets=1  coefficient_reload=off  filter_type=Single_Rate  rate_change_type=Integer  interpolation_rate=1  decimation_rate=1  zero_pack_factor=1  channel_sequence=Basic  number_channels=1  pattern_list='P4-0,P4-1,P4-2,P4-3,P4-4'  number_paths=1  ratespecification=Maximum_Possible  sampleperiod=12  hardwareoversamplingrate=1  coefficient_sign=Signed  quantization=Quantize_Only  coefficient_width=16  bestprecision=off  coefficient_fractional_bits=15  coefficient_structure=Inferred  output_rounding_mode=Truncate_LSBs  output_width=18  filter_architecture=Systolic_Multiply_Accumulate  optimization_goal=Area  optimization_list='None'  data_buffer_type=Automatic  coefficient_buffer_type=Automatic  input_buffer_type=Automatic  output_buffer_type=Automatic  preference_for_other_storage=Automatic  multi_column_support=Automatic  columnconfig='8'  inter_column_pipe_length=4  data_has_tlast=Not_Required  m_data_has_tready=off  s_data_has_fifo=off  s_data_has_tuser=Not_Required  m_data_has_tuser=Not_Required  s_config_sync_mode=On_Vector  s_config_method=Single  num_reload_slots=1  has_aclken=off  has_aresetn=off  infoeditControl=ARESETn must be asserted for a minimum of 2 cycles  reset_data_vector=on  trim_axipin_name=on  simulation_type=hybrid_sim  simulation_model=sysgen:xfirv7_2_cmodel  data_path_portlist={ 's_axis_data_tdata', 'm_axis_data_tdata' }  passband_min=0.0  passband_max=0.5  stopband_min=0.5  stopband_max=1.0  filter_selection=1  gui_behaviour='Sysgen_GUI'  data_sign=Signed  data_width=16  data_fractional_bits=0  data_tuser_width=1  wrapper_available=true  ip_wrap_arbitrary_binary_point=true  ip_name=FIR Compiler  ip_version=7.2  dsptool_ready=true  ipcore_usecache=true  ipcore_useipmodelcache=true  port_translation_map={ 'aclken' => 'en', 'aresetn' => 'rst' }  run_core_at_system_period=true  ipcore_xco_need_fpga_part=true  block_type=fir_compiler_v7_2
      settings: infoedit=Maximum Possible : Maximizes oversampling rate. Abstracted input handshake (no s_data_tvalid) and automatic rate propagation.<br>Hardware Oversampling Rate : Specifies oversampling rate relative to the input sample period. Abstracted input handshake (no s_data_tvalid) and automatic rate propagation.<br>Input/Output Sample Period : Specifies absolute oversampling rate. No input handshake abstraction (exposes s_data_tvalid) and no rate propagation.
  Gateway Out{3..5,7} (4 alike) : xbsIndex_r4/Gateway Out  inherit_from_input=off  hdl_port=off  rows=1  columns=1  UseAsDAC=off  DACChannel='1'  interface=None  automatic_assignment=on  address_offset=hex2dec('00')  intf_name=''  intf_description=''  timing_constraint=None  locs_specified=off  LOCs={}  io_standard={}  block_type=gatewayout
  Scope4 : Scope  NumInputPorts=4
  four_point_avg : Subsystem
  Window_profile : Outport
  filtered_Q : Outport  Port=2
  filtered_I : Outport  Port=3
  wires:
  [window] -> Gateway Out3/1
  "CORDIC 6.0 "/2 -> Gateway Out5/1
  eval_window/1 -> [window]
  [c1p2_pt_cntr] -> Gateway Out7/1
  Gateway Out5/1 -> Scope4/2
  real/1 -> FIR Compiler 7.2 2/1
  [cav1_p2_dc_tvalid] -> "CORDIC 6.0 "/1
  four_point_avg/1(Out1) -> Window_profile/1
  "CORDIC 6.0 "/3 -> four_point_avg/1(In1), Gateway Out4/1
  FIR Compiler 7.2 2/3 -> filtered_I/1, "CORDIC 6.0 "/3
  imag/1 -> FIR Compiler 7.2 3/1
  FIR Compiler 7.2 3/3 -> filtered_Q/1, "CORDIC 6.0 "/2
  Gateway Out4/1 -> Scope4/1
  Gateway Out7/1 -> Scope4/3
  Gateway Out3/1 -> Scope4/4

== system exampleModel_bus_axi_w_4ptavg/example/dsp/Cav2/DDC NCO1 ==
  Phase_ctrl : Inport
  Phase_reset : Inport  Port=2
  Bus Creator : BusCreator  Inputs=2
  Constant21 : xbsIndex_r4/Constant  const=1  gui_display_data_type=Boolean  arith_type=Boolean  n_bits=4  bin_pt=0  preci_type=Single  exp_width=8  frac_width=24  explicit_period=on  period=1/Fsig  equ=P=C  opselect=C  inp2=PCIN>>17  opr=+  inp1=P  carry=CIN  dbl_ovrd=off  block_type=constant
  Convert : xbsIndex_r4/Convert  gui_display_data_type=Boolean  arith_type=Boolean  n_bits=16  bin_pt=14  float_type=Single  exp_bits=8  fraction_bits=24  quantization=Truncate  overflow=Wrap  en=off  latency=1  pipeline=off  dbl_ovrd=off  block_type=convert
  "DDS Compiler 6.0 " : xbsIndex_r4/DDS Compiler 6.0   partspresent=Phase_Generator_and_SIN_COS_LUT  dds_clock_rate=17  channels=1  mode_of_operation=Standard  modulus=9  parameter_entry=Hardware_Parameters  spurious_free_dynamic_range=45  frequency_resolution=0.4  noise_shaping=Taylor_Series_Corrected  phase_width=32  output_width=26  output_selection=Sine_and_Cosine  negative_sine=off  negative_cosine=off  amplitude_mode=Unit_Circle  memory_type=Auto  optimization_goal=Auto  dsp48_use=Minimal  resync=on  latency_configuration=Auto  latency=1  has_phase_out=off  has_aclken=off  has_aresetn=off  explicit_period=off  period=1/Fproc  data_has_tlast=Not_Required  has_tready=on  s_phase_has_tuser=Not_Required  m_data_has_tuser=Not_Required  m_phase_has_tuser=Not_Required  s_phase_tuser_width=1  output_form=Twos_Complement  s_config_sync_mode=On_Vector  phase_increment=Streaming  output_frequency1=0  output_frequency2=0  output_frequency3=0  output_frequency4=0  output_frequency5=0  output_frequency6=0  output_frequency7=0  output_frequency8=0  output_frequency9=0  output_frequency10=0  output_frequency11=0  output_frequency12=0  output_frequency13=0  output_frequency14=0  output_frequency15=0  output_frequency16=0  pinc1='0'  pinc2='0'  pinc3='0'  pinc4='0'  pinc5='0'  pinc6='0'  pinc7='0'  pinc8='0'  pinc9='0'  pinc10='0'  pinc11='0'  pinc12='0'  pinc13='0'  pinc14='0'  pinc15='0'  pinc16='0'  phase_offset=None  phase_offset_angles1=0  phase_offset_angles2=0  phase_offset_angles3=0  phase_offset_angles4=0  phase_offset_angles5=0  phase_offset_angles6=0  phase_offset_angles7=0  phase_offset_angles8=0  phase_offset_angles9=0  phase_offset_angles10=0  phase_offset_angles11=0  phase_offset_angles12=0  phase_offset_angles13=0  phase_offset_angles14=0  phase_offset_angles15=0  phase_offset_angles16=0  poff1='0'  poff2='0'  poff3='0'  poff4='0'  poff5='0'  poff6='0'  poff7='0'  poff8='0'  poff9='0'  poff10='0'  poff11='0'  poff12='0'  poff13='0'  poff14='0'  poff15='0'  poff16='0'  trim_axipin_name=off  simulation_type=hybrid_sim  simulation_model=sysgen:xddsv6_0_cmodel  data_path_portlist={ 's_axis_config_tdata_poff', 's_axis_config_tdata_chan0_poff', 's_axis_config_tdata_pinc', 's_axis_config_tdata_chan0_pinc', 's_axis_phase_tdata_resync', 's_axis_phase_tdata_chan0_resync', 's_axis_phase_tdata_poff', 's_axis_phase_tdata_chan0_poff', 's_axis_phase_tdata_pinc', 's_axis_phase_tdata_chan0_pinc', 's_axis_phase_tdata_phase_in', 'm_axis_data_tdata_sine', 'm_axis_data_tdata_chan0_sine', 'm_axis_data_tdata_cosine', 'm_axis_data_tdata_chan0_cosine', 'm_axis_phase_tdata_phase_out', 'm_axis_phase_tdata_chan0_phase_out'}  por_mode=false  gui_behaviour=Sysgen  ip_name=DDS Compiler  ip_version=6.0  dsptool_ready=true  wrapper_available=true  port_translation_map={ 'aclken' => 'en', 'aresetn' => 'rst' }  ipcore_usecache=true  ipcore_useipmodelcache=true  ipcore_xco_need_fpga_part=true  ipcore_verbose=false  block_type=dds_compiler_v6_0
  Logical : xbsIndex_r4/Logical  logical_function=NAND  inputs=2  en=off  latency=1  precision=Full  arith_type=Unsigned  n_bits=16  bin_pt=0  align_bp=on  dbl_ovrd=off  block_type=logical
  posedge_pulse : Subsystem
  tvalid : Outport
  Out2 : Outport  Port=2
  Sine : Outport  Port=3
  Cosine : Outport  Port=4
  NCO_out : Outport  Port=5
  wires:
  "DDS Compiler 6.0 "/1 -> Out2/1
  Constant21/1 -> Logical/1
  Bus Creator/1 -> NCO_out/1
  "DDS Compiler 6.0 "/3 -> Bus Creator/1, Sine/1  "NCO_sin"
  "DDS Compiler 6.0 "/4 -> Bus Creator/2, Cosine/1  "NCO_cos"
  "DDS Compiler 6.0 "/2 -> tvalid/1
  Phase_reset/1 -> posedge_pulse/1(In1)
  Logical/1 -> "DDS Compiler 6.0 "/4, "DDS Compiler 6.0 "/1
  Convert/1 -> Logical/2
  posedge_pulse/1(Out1) -> "DDS Compiler 6.0 "/2, Convert/1
  Phase_ctrl/1 -> "DDS Compiler 6.0 "/3

== system exampleModel_bus_axi_w_4ptavg/example/dsp/Cav2/IQ_integration ==
  cav_windowed_imag : Inport
  cav_windowed_real : Inport  Port=2
  ref_windowed_i : Inport  Port=3
  ref_windowed_q : Inport  Port=4
  window_profile : Inport  Port=5
  Accumulator{,1..3} (4 alike) : xbsIndex_r4/Accumulator  operation=Add  n_bits=32  overflow=Wrap  scale=1  rst=on  hasbypass=off  infoeditControl=reset for floating point data type must be asserted for a minimum of 2 cycles  en=off  latency=1  msb_inp=100  msb=100  lsb=-100  use_behavioral_HDL=on  implementation=Fabric  dbl_ovrd=off  block_type=accum
  Convert{1,3,5..6} (4 alike) : xbsIndex_r4/Convert  gui_display_data_type=Boolean  arith_type=Boolean  n_bits=16  bin_pt=14  float_type=Single  exp_bits=8  fraction_bits=24  quantization=Truncate  overflow=Wrap  en=off  latency=1  pipeline=off  dbl_ovrd=off  block_type=convert
  Convert{2,4,9..10} (4 alike) : xbsIndex_r4/Convert  gui_display_data_type=Fixed-point  arith_type="Signed  (2's comp)"  n_bits=20  bin_pt=18  float_type=Single  exp_bits=8  fraction_bits=24  quantization=Truncate  overflow=Wrap  en=off  latency=1  pipeline=off  dbl_ovrd=off  block_type=convert
  Display{1..8} (8 alike) : Display
  Gateway Out{,1..18,22..23} (21 alike) : xbsIndex_r4/Gateway Out  inherit_from_input=off  hdl_port=on  rows=1  columns=1  UseAsDAC=off  DACChannel='1'  interface=None  automatic_assignment=on  address_offset=hex2dec('00')  intf_name=''  intf_description=''  timing_constraint=None  locs_specified=off  LOCs={}  io_standard={}  block_type=gatewayout
  Inverter{,1..3} (4 alike) : xbsIndex_r4/Inverter  en=off  latency=1  dbl_ovrd=off  block_type=inv
  Register{1..2,11..12} (4 alike) : xbsIndex_r4/Register  init=0  rst=off  en=on  dbl_ovrd=off  block_type=register
  Scope{1..9} (9 alike) : Scope  NumInputPorts=3
  cav_int_q : Outport
  cav_int_i : Outport  Port=2
  ref_int_i : Outport  Port=3
  ref_int_q : Outport  Port=4
  wires:
  Gateway Out13/1 -> Display2/1, Scope6/2
  Gateway Out6/1 -> Scope3/3, Scope7/3
  Accumulator1/1 -> Register11/1, Gateway Out7/1
  cav_windowed_real/1 -> Accumulator1/1, Gateway Out8/1
  Gateway Out/1 -> Scope6/3, Scope2/3
  Convert6/1 -> Register11/2, Inverter1/1
  [window] -> Convert5/1
  Convert5/1 -> Register12/2, Inverter/1
  Gateway Out8/1 -> Scope3/1, Scope7/1
  Accumulator/1 -> Register12/1, Gateway Out3/1
  Gateway Out9/1 -> Display1/1, Scope7/2
  Gateway Out3/1 -> Scope2/2
  Gateway Out5/1 -> Scope6/1, Scope2/1
  [window] -> Convert6/1
  Inverter/1 -> Gateway Out/1, Accumulator/2
  cav_windowed_imag/1 -> Gateway Out5/1, Accumulator/1
  Gateway Out7/1 -> Scope3/2
  Gateway Out23/1 -> Display4/1
  Gateway Out22/1 -> Display3/1
  Inverter1/1 -> Accumulator1/2, Gateway Out6/1
  Inverter2/1 -> Gateway Out2/1, Accumulator2/2
  Gateway Out1/1 -> Scope9/3, Display6/1
  Gateway Out4/1 -> Scope1/2
  [window] -> Convert1/1
  Gateway Out11/1 -> Scope9/1, Scope4/2, Display5/1
  Gateway Out10/1 -> Scope4/1, Scope1/1
  Convert1/1 -> Register1/2, Inverter2/1
  ref_windowed_i/1 -> Gateway Out10/1, Accumulator2/1
  Accumulator2/1 -> Gateway Out4/1, Register1/1
  Gateway Out2/1 -> Scope4/3, Scope1/3
  Gateway Out16/1 -> Scope5/3, Scope8/3
  Accumulator3/1 -> Register2/1, Gateway Out17/1
  ref_windowed_q/1 -> Accumulator3/1, Gateway Out14/1
  Convert3/1 -> Register2/2, Inverter3/1
  Gateway Out14/1 -> Scope5/1, Scope8/1
  Gateway Out15/1 -> Display7/1, Scope8/2
  [window] -> Convert3/1
  Gateway Out17/1 -> Scope5/2
  Gateway Out12/1 -> Display8/1
  Inverter3/1 -> Accumulator3/2, Gateway Out16/1
  Convert9/1 -> Gateway Out22/1, cav_int_i/1
  Convert10/1 -> cav_int_q/1, Gateway Out23/1
  Convert2/1 -> ref_int_i/1, Gateway Out1/1
  Convert4/1 -> ref_int_q/1, Gateway Out12/1
  window_profile/1 -> [window]
  Register1/1 -> Gateway Out18/1, Convert2/1, Gateway Out11/1
  Gateway Out18/1 -> Scope9/2
  Register2/1 -> Convert4/1, Gateway Out15/1
  Register11/1 -> Convert9/1, Gateway Out9/1
  Register12/1 -> Convert10/1, Gateway Out13/1
